simulink model "DC_MOTOR"  (R2020a)
settings: Solver=VariableStepAuto  StartTime=0.0  StopTime=10.0  RelTol=1e-3
settings Model: Creator=raghu  LastModifiedBy=raghu

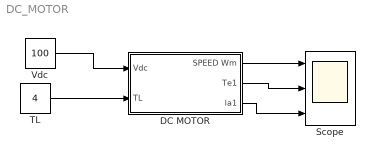
== system DC_MOTOR ==
  DC MOTOR : Subsystem
  Scope : Scope  NumInputPorts=3
  TL : Constant  Value=4
  Vdc : Constant  Value=100
  wires:
  Vdc/1 -> DC MOTOR/1(Vdc)
  TL/1 -> DC MOTOR/2(TL)
  DC MOTOR/2(Te1) -> Scope/2
  DC MOTOR/1(SPEED Wm) -> Scope/1
  DC MOTOR/3(la1) -> Scope/3

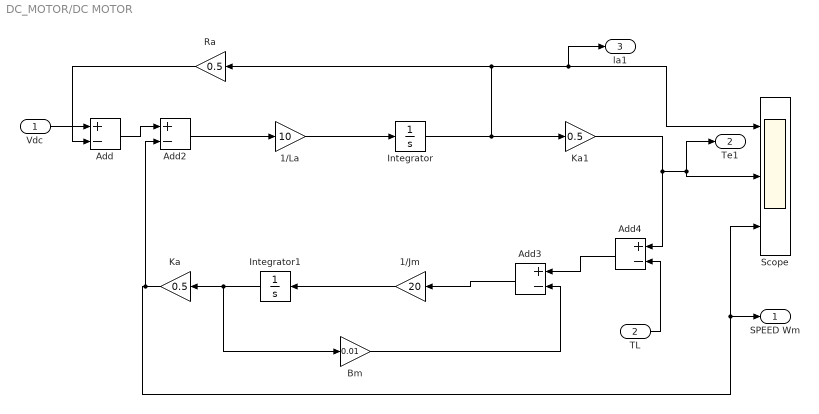
== system DC_MOTOR/DC MOTOR ==
  Vdc : Inport
  TL : Inport  Port=2
  1/Jm : Gain  Gain=20
  1/La : Gain  Gain=10
  Add{,2..4} (4 alike) : Sum  Inputs=+-
  Bm : Gain  Gain=0.01
  Integrator : Integrator
  Integrator1 : Integrator
  Ka : Gain  Gain=0.5
  Ka1 : Gain  Gain=0.5
  Ra : Gain  Gain=0.5
  Scope : Scope  NumInputPorts=3
  SPEED Wm : Outport
  Te1 : Outport  Port=2
  la1 : Outport  Port=3
  wires:
  TL/1 -> Add4/2
  Ka/1 -> SPEED Wm/1, Scope/3, Add2/2
  Ra/1 -> Add/2
  1/Jm/1 -> Integrator1/1
  Integrator/1 -> Scope/1, la1/1, Ra/1, Ka1/1
  Add/1 -> Add2/1
  Ka1/1 -> Add4/1, Te1/1, Scope/2
  Add2/1 -> 1/La/1
  Integrator1/1 -> Bm/1, Ka/1
  Vdc/1 -> Add/1
  1/La/1 -> Integrator/1
  Add4/1 -> Add3/1
  Bm/1 -> Add3/2
  Add3/1 -> 1/Jm/1
